simulink model "scpi_sim2"  (R2024b)
settings: Solver=VariableStepAuto  StartTime=0.0  StopTime=50  RelTol=1e-3
values from neighbouring files (symbols this model uses):
  H2 = 0.06/(0.206*s+1)/(0.24*s+1)/(12*s+1)*exp(-0.2*s)    [SCPI.m]
  Kr2 = 20.4    [SCPI.m]
  Td2 = 0.235    [SCPI.m]
  Ti2 = 12.24    [SCPI.m]
settings Model: Creator=Student  LastModifiedBy=mihne
settings SolverCC: AlgebraicLoopSolver=TrustRegion
settings DebuggingCC: UnconnectedInputMsg=warning  UnconnectedOutputMsg=warning  UnconnectedLineMsg=warning
settings ModelReferenceCC: EnableRefExpFcnMdlSchedulingChecks=on
settings RTWCC: GPUComputeCapability=3.5  DLArmComputeVersion=19.05

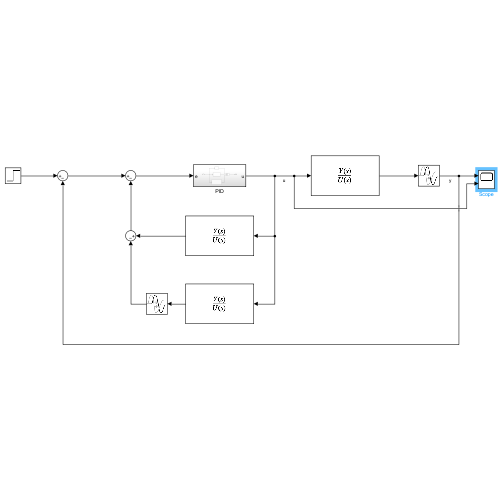
[thumbnail: Simulink's stored preview of the top-level diagram]
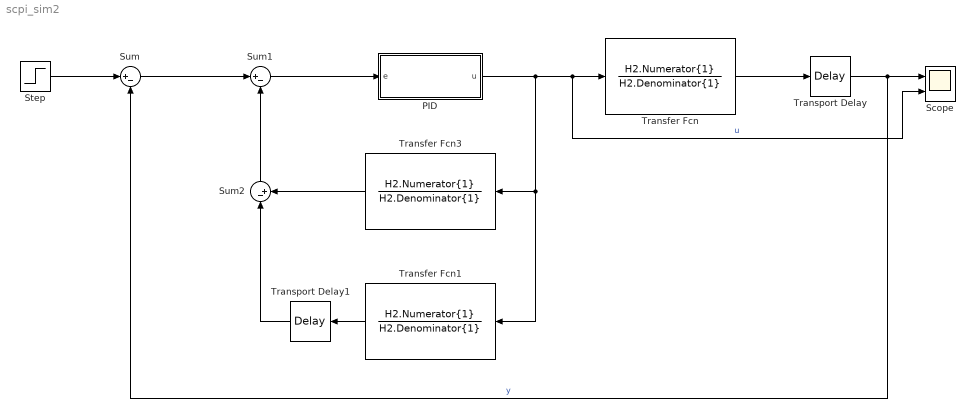
== system scpi_sim2 ==
  PID : Subsystem
  Scope : Scope  NumInputPorts=2
  Step : Step  Time=0  After=5  SampleTime=0
  Sum : Sum  Inputs=|+-
  Sum1 : Sum  Inputs=|+-
  Sum2 : Sum  Inputs=|-+
  Transfer Fcn : TransferFcn  Numerator=H2.Numerator{1}  Denominator=H2.Denominator{1}
  Transfer Fcn1 : TransferFcn  Numerator=H2.Numerator{1}  Denominator=H2.Denominator{1}
  Transfer Fcn3 : TransferFcn  Numerator=H2.Numerator{1}  Denominator=H2.Denominator{1}
  Transport Delay : TransportDelay  DelayTime=0.2
  Transport Delay1 : TransportDelay  DelayTime=0.2
  wires:
  Step/1 -> Sum/1
  Transfer Fcn/1 -> Transport Delay/1
  Transport Delay1/1 -> Sum2/1
  Transfer Fcn1/1 -> Transport Delay1/1
  Transfer Fcn3/1 -> Sum2/2
  Transport Delay/1 -> Sum/2, Scope/1  "y"
  Sum2/1 -> Sum1/2
  PID/1(u) -> Transfer Fcn3/1, Transfer Fcn1/1, Scope/2, Transfer Fcn/1  "u"
  Sum/1 -> Sum1/1
  Sum1/1 -> PID/1(e)

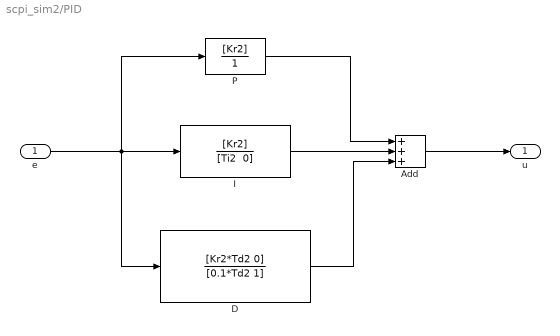
== system scpi_sim2/PID ==
  e : Inport
  Add : Sum  Inputs=+++
  D : TransferFcn  Numerator=[Kr2*Td2 0]  Denominator=[0.1*Td2 1]
  I : TransferFcn  Numerator=[Kr2]  Denominator="[Ti2  0]"
  P : TransferFcn  Numerator=[Kr2]  Denominator=[1]
  u : Outport
  wires:
  e/1 -> P/1, I/1, D/1
  Add/1 -> u/1
  P/1 -> Add/1
  D/1 -> Add/3
  I/1 -> Add/2
